simulink model "Adaptive_Noise"  (R2015a)
settings: Solver=ode45  StartTime=0.0  StopTime=5  RelTol=1e-3
libraries: dspadpt3 x1
settings Model: Creator=yuzhouliu  LastModifiedBy=yuzhouliu
settings SolverCC: AlgebraicLoopSolver=LineSearch

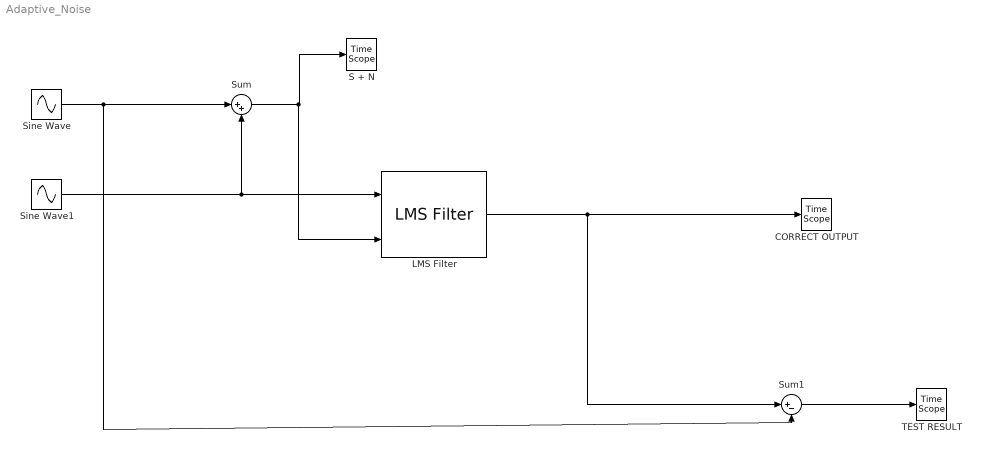
== system Adaptive_Noise ==
  CORRECT OUTPUT : TimeScope  DefaultConfigurationName=spbscopes.TimeScopeBlockCfg
  LMS Filter : dspadpt3/LMS Filter  Algo=LMS  L=20  stepflag=Dialog  mu=0.002  leakage=1.0  ic=0.02  Adapt=off  resetflag=None  weights=on  secondCoeffMode=User-defined  secondCoeffWordLength=2  secondCoeffFracLength=15  accum2Mode=User-defined  accum2FracLength=20  prodOutput2Mode=User-defined  prodOutput2FracLength=20  prodOutput3Mode=User-defined  prodOutput3FracLength=20  prodOutput4Mode=User-defined  prodOutput4FracLength=20  quotientMode=User-defined  quotientFracLength=20  roundingMode=Floor  overflowMode=off  addnparflag=off
  S + N : TimeScope  DefaultConfigurationName=spbscopes.TimeScopeBlockCfg
  Sine Wave : Sin  Frequency=2*pi*200  SampleTime=0.00001
  Sine Wave1 : Sin  Frequency=2*pi*60  SampleTime=0.0001
  Sum : Sum  Inputs=|++
  Sum1 : Sum  Inputs=|+-
  TEST RESULT : TimeScope  DefaultConfigurationName=spbscopes.TimeScopeBlockCfg
  wires:
  Sine Wave/1 -> Sum1/2, Sum/1
  Sine Wave1/1 -> LMS Filter/1, Sum/2
  Sum/1 -> LMS Filter/2, S + N/1
  LMS Filter/2 -> Sum1/1, CORRECT OUTPUT/1
  Sum1/1 -> TEST RESULT/1
